simulink library "sldvdemo_custom_blockreplib_R2010b"  (Simulink 7.6)
settings: Solver=ode45  SolverMode=SingleTasking  StartTime=0.0  StopTime=10.0  RelTol=1e-3
libraries: sldvlib x1
settings Model: Creator=The MathWorks Inc.  LastModifiedBy=itoy  ExtModeAutoUpdateStatusClock=off

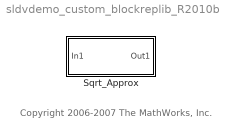
== system sldvdemo_custom_blockreplib_R2010b ==
  note: Copyright 2006-2007 The MathWorks, Inc.
  Sqrt_Approx : Subsystem  mask(SldvDemo  Math Function-Sqrt  Replacement){OutMin=[], OutMax=[], OutDataTypeStr=double}
      mask prompts: OutMin "Output minimum:"; OutMax "Output maximum:"; OutDataTypeStr "Output data type:"
      mask help: Approximates the mathematical function sqrt using lookup table. The input range is constrained to [0 10000].
      mask init:
      | xdata = [0.00 1.00 6.88 25.57 68.58 150.80 291.27 512.11 ...
      |          839.14 1302.55 1935.79 2775.50 3862.12 5240.99 ...
      |          6959.23 9069.32 10000.00];
      | 
      | ydata = [0.00 1.00 2.62 5.06 8.28 12.28 17.07 22.63 28.97 ...                              
      |          36.09 44.00 52.68 62.15 72.39 83.42 95.23 100.00];
      | 
      | maskOutMin = get_param(gcb,'OutMin');
      | maskOutMax = get_param(gcb,'OutMax');
      | maskOutDataTypeStr = get_param(gcb,'OutDataTypeStr');
      | 
      | targetBlock = [gcb '/Lookup Table'];
      | 
      | set_param(targetBlock,'OutMin',maskOutMin);
      | set_param(targetBlock,'OutMax',maskOutMax);
      | set_param(targetBlock,'OutDataTypeStr',maskOutDataTypeStr);
      mask Help: Approximates the mathematical function sqrt using lookup table. The input range is constrained to [0 10000].
      mask StyleString: edit,edit,popup(Inherit: Inherit via back propagation|Inherit: Same as input|double|single)
      mask Display:
      | disp('sqrt');
      | port_label('input',1,'C');

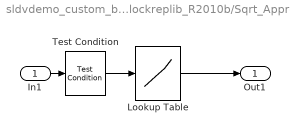
== system sldvdemo_custom_blockreplib_R2010b/Sqrt_Approx ==
  In1 : Inport
  Lookup Table : Lookup  InputValues=xdata  Table=ydata  LookUpMeth=Interpolation-Use End Values  OutDataTypeStr=double
  Test Condition : sldvlib/Test Condition  SystemSampleTime=-1  enabled=on  customAVTBlockType=Test Condition  intervals={[0, 10000]}  initial=off  dispValues=on  outEnabled=on
      settings: AttributesFormatString=%<intervals>
  Out1 : Outport
  wires:
  In1/1 -> Test Condition/1
  Lookup Table/1 -> Out1/1
  Test Condition/1 -> Lookup Table/1
